simulink model "External_Light"  (R2020b)
settings: Solver=VariableStepAuto  StartTime=0.0  StopTime=10.0  RelTol=1e-3
settings Model: Creator=training  LastModifiedBy=training

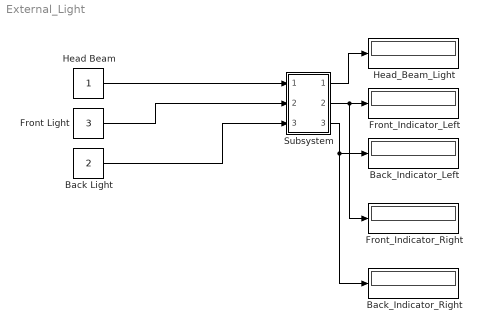
== system External_Light ==
  Back Light : Constant  Value=2
  Back_Indicator_Left : Display
  Back_Indicator_Right : Display
  Front Light : Constant  Value=3
  Front_Indicator_Left : Display
  Front_Indicator_Right : Display
  Head Beam : Constant
  Head_Beam_Light : Display
  Subsystem : Subsystem
  wires:
  Head Beam/1 -> Subsystem/1(In1)
  Front Light/1 -> Subsystem/2(In2)
  Subsystem/1(Out1) -> Head_Beam_Light/1
  Subsystem/2(Out2) -> Front_Indicator_Right/1, Front_Indicator_Left/1
  Subsystem/3(Out3) -> Back_Indicator_Right/1, Back_Indicator_Left/1
  Back Light/1 -> Subsystem/3(In3)

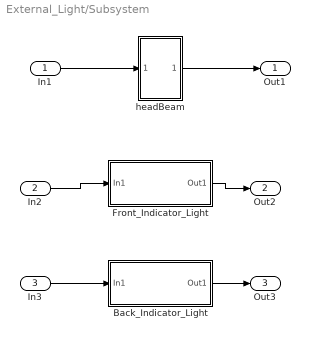
== system External_Light/Subsystem ==
  In1 : Inport
  In2 : Inport  Port=2
  In3 : Inport  Port=3
  Back_Indicator_Light : Subsystem  Variant=on
  Front_Indicator_Light : Subsystem  Variant=on
  headBeam : Subsystem
  Out1 : Outport
  Out2 : Outport  Port=2
  Out3 : Outport  Port=3
  wires:
  Back_Indicator_Light/1(Out1) -> Out3/1
  In1/1 -> headBeam/1(In1)
  In2/1 -> Front_Indicator_Light/1(In1)
  Front_Indicator_Light/1(Out1) -> Out2/1
  headBeam/1(Out1) -> Out1/1
  In3/1 -> Back_Indicator_Light/1(In1)

== system External_Light/Subsystem/Back_Indicator_Light ==
  note: 1) Add Subsystem or Model blocks as valid variant choices.
      | 2) You cannot connect blocks at this level. At simulation, connectivity is automatically
      | determined, based on the active variant and port name matching.
  In1 : Inport
  Back_Indicator_Left : Subsystem  VariantControl=Choice_1
  Back_Indicator_Right : Subsystem  VariantControl=Choice_2
  Out1 : Outport

== system External_Light/Subsystem/Front_Indicator_Light ==
  note: 1) Add Subsystem or Model blocks as valid variant choices.
      | 2) You cannot connect blocks at this level. At simulation, connectivity is automatically
      | determined, based on the active variant and port name matching.
  In1 : Inport
  Front_Indicator_Left : Subsystem  VariantControl=Choice_1
  Front_Indicator_Right : Subsystem  VariantControl=Choice_2
  Out1 : Outport

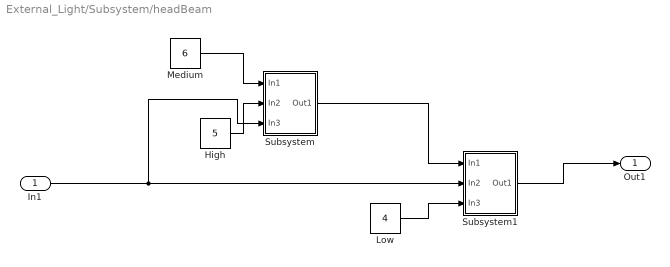
== system External_Light/Subsystem/headBeam ==
  In1 : Inport
  High : Constant  Value=5
  Low : Constant  Value=4
  Medium : Constant  Value=6
  Subsystem : Subsystem
  Subsystem1 : Subsystem
  Out1 : Outport
  wires:
  High/1 -> Subsystem/2(In2)
  Subsystem/1(Out1) -> Subsystem1/1(In1)
  Medium/1 -> Subsystem/1(In1)
  In1/1 -> Subsystem/3(In3), Subsystem1/2(In2)
  Low/1 -> Subsystem1/3(In3)
  Subsystem1/1(Out1) -> Out1/1

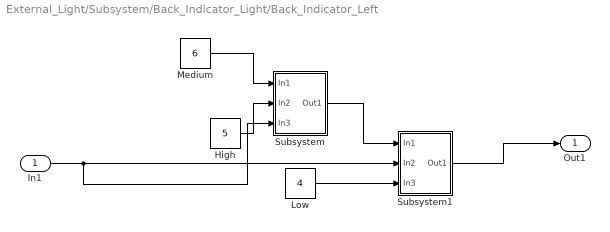
== system External_Light/Subsystem/Back_Indicator_Light/Back_Indicator_Left ==
  In1 : Inport
  High : Constant  Value=5
  Low : Constant  Value=4
  Medium : Constant  Value=6
  Subsystem : Subsystem
  Subsystem1 : Subsystem
  Out1 : Outport
  wires:
  In1/1 -> Subsystem/3(In3), Subsystem1/2(In2)
  Subsystem1/1(Out1) -> Out1/1
  Subsystem/1(Out1) -> Subsystem1/1(In1)
  High/1 -> Subsystem/2(In2)
  Medium/1 -> Subsystem/1(In1)
  Low/1 -> Subsystem1/3(In3)

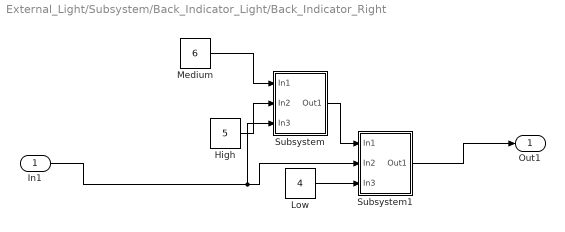
== system External_Light/Subsystem/Back_Indicator_Light/Back_Indicator_Right ==
  In1 : Inport
  High : Constant  Value=5
  Low : Constant  Value=4
  Medium : Constant  Value=6
  Subsystem : Subsystem
  Subsystem1 : Subsystem
  Out1 : Outport
  wires:
  Low/1 -> Subsystem1/3(In3)
  Subsystem/1(Out1) -> Subsystem1/1(In1)
  High/1 -> Subsystem/2(In2)
  In1/1 -> Subsystem/3(In3), Subsystem1/2(In2)
  Subsystem1/1(Out1) -> Out1/1
  Medium/1 -> Subsystem/1(In1)

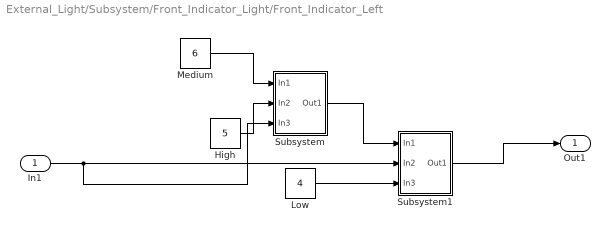
== system External_Light/Subsystem/Front_Indicator_Light/Front_Indicator_Left ==
  In1 : Inport
  High : Constant  Value=5
  Low : Constant  Value=4
  Medium : Constant  Value=6
  Subsystem : Subsystem
  Subsystem1 : Subsystem
  Out1 : Outport
  wires:
  In1/1 -> Subsystem/3(In3), Subsystem1/2(In2)
  Subsystem1/1(Out1) -> Out1/1
  Subsystem/1(Out1) -> Subsystem1/1(In1)
  High/1 -> Subsystem/2(In2)
  Medium/1 -> Subsystem/1(In1)
  Low/1 -> Subsystem1/3(In3)

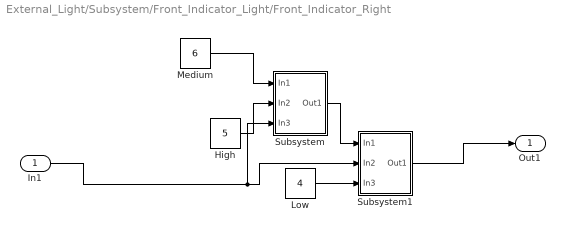
== system External_Light/Subsystem/Front_Indicator_Light/Front_Indicator_Right ==
  In1 : Inport
  High : Constant  Value=5
  Low : Constant  Value=4
  Medium : Constant  Value=6
  Subsystem : Subsystem
  Subsystem1 : Subsystem
  Out1 : Outport
  wires:
  Low/1 -> Subsystem1/3(In3)
  Subsystem/1(Out1) -> Subsystem1/1(In1)
  High/1 -> Subsystem/2(In2)
  In1/1 -> Subsystem/3(In3), Subsystem1/2(In2)
  Subsystem1/1(Out1) -> Out1/1
  Medium/1 -> Subsystem/1(In1)

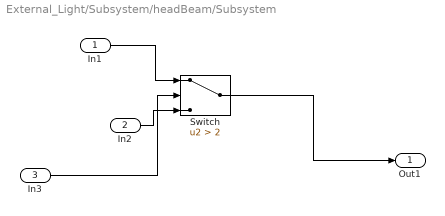
== system External_Light/Subsystem/headBeam/Subsystem ==
  In1 : Inport
  In2 : Inport  Port=2
  In3 : Inport  Port=3
  Switch : Switch  Criteria=u2 > Threshold  Threshold=2
  Out1 : Outport
  wires:
  In3/1 -> Switch/2
  Switch/1 -> Out1/1
  In1/1 -> Switch/1
  In2/1 -> Switch/3

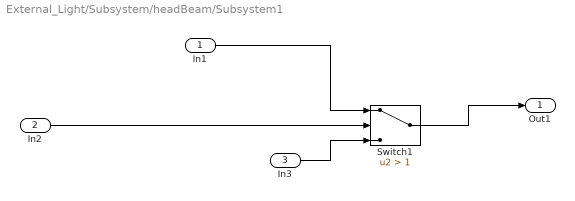
== system External_Light/Subsystem/headBeam/Subsystem1 ==
  In1 : Inport
  In2 : Inport  Port=2
  In3 : Inport  Port=3
  Switch1 : Switch  Criteria=u2 > Threshold  Threshold=1
  Out1 : Outport
  wires:
  In1/1 -> Switch1/1
  Switch1/1 -> Out1/1
  In3/1 -> Switch1/3
  In2/1 -> Switch1/2

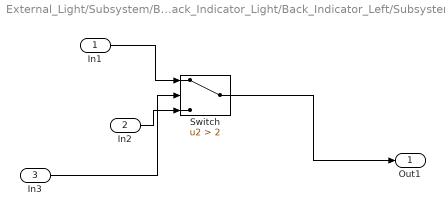
== system External_Light/Subsystem/Back_Indicator_Light/Back_Indicator_Left/Subsystem ==
  In1 : Inport
  In2 : Inport  Port=2
  In3 : Inport  Port=3
  Switch : Switch  Criteria=u2 > Threshold  Threshold=2
  Out1 : Outport
  wires:
  In3/1 -> Switch/2
  Switch/1 -> Out1/1
  In1/1 -> Switch/1
  In2/1 -> Switch/3

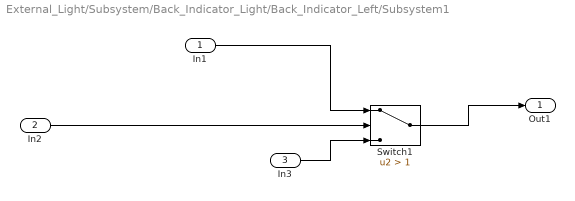
== system External_Light/Subsystem/Back_Indicator_Light/Back_Indicator_Left/Subsystem1 ==
  In1 : Inport
  In2 : Inport  Port=2
  In3 : Inport  Port=3
  Switch1 : Switch  Criteria=u2 > Threshold  Threshold=1
  Out1 : Outport
  wires:
  In1/1 -> Switch1/1
  Switch1/1 -> Out1/1
  In3/1 -> Switch1/3
  In2/1 -> Switch1/2

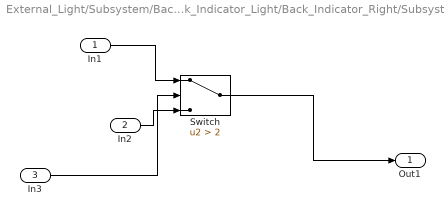
== system External_Light/Subsystem/Back_Indicator_Light/Back_Indicator_Right/Subsystem ==
  In1 : Inport
  In2 : Inport  Port=2
  In3 : Inport  Port=3
  Switch : Switch  Criteria=u2 > Threshold  Threshold=2
  Out1 : Outport
  wires:
  In3/1 -> Switch/2
  Switch/1 -> Out1/1
  In1/1 -> Switch/1
  In2/1 -> Switch/3

== system External_Light/Subsystem/Back_Indicator_Light/Back_Indicator_Right/Subsystem1 ==
  In1 : Inport
  In2 : Inport  Port=2
  In3 : Inport  Port=3
  Switch1 : Switch  Criteria=u2 > Threshold  Threshold=1
  Out1 : Outport
  wires:
  In1/1 -> Switch1/1
  Switch1/1 -> Out1/1
  In3/1 -> Switch1/3
  In2/1 -> Switch1/2

== system External_Light/Subsystem/Front_Indicator_Light/Front_Indicator_Left/Subsystem ==
  In1 : Inport
  In2 : Inport  Port=2
  In3 : Inport  Port=3
  Switch : Switch  Criteria=u2 > Threshold  Threshold=2
  Out1 : Outport
  wires:
  In3/1 -> Switch/2
  Switch/1 -> Out1/1
  In1/1 -> Switch/1
  In2/1 -> Switch/3

== system External_Light/Subsystem/Front_Indicator_Light/Front_Indicator_Left/Subsystem1 ==
  In1 : Inport
  In2 : Inport  Port=2
  In3 : Inport  Port=3
  Switch1 : Switch  Criteria=u2 > Threshold  Threshold=1
  Out1 : Outport
  wires:
  In1/1 -> Switch1/1
  Switch1/1 -> Out1/1
  In3/1 -> Switch1/3
  In2/1 -> Switch1/2

== system External_Light/Subsystem/Front_Indicator_Light/Front_Indicator_Right/Subsystem ==
  In1 : Inport
  In2 : Inport  Port=2
  In3 : Inport  Port=3
  Switch : Switch  Criteria=u2 > Threshold  Threshold=2
  Out1 : Outport
  wires:
  In3/1 -> Switch/2
  Switch/1 -> Out1/1
  In1/1 -> Switch/1
  In2/1 -> Switch/3

== system External_Light/Subsystem/Front_Indicator_Light/Front_Indicator_Right/Subsystem1 ==
  In1 : Inport
  In2 : Inport  Port=2
  In3 : Inport  Port=3
  Switch1 : Switch  Criteria=u2 > Threshold  Threshold=1
  Out1 : Outport
  wires:
  In1/1 -> Switch1/1
  Switch1/1 -> Out1/1
  In3/1 -> Switch1/3
  In2/1 -> Switch1/2
